simulink model "course_loop"  (R2019a)
settings: Solver=VariableStepAuto  StartTime=0.0  StopTime=300  RelTol=1e-3
undefined symbols (not defined in the file or in its folder): AP, trans_func
settings Model: Creator=nikhil  LastModifiedBy=VTOL_HYD

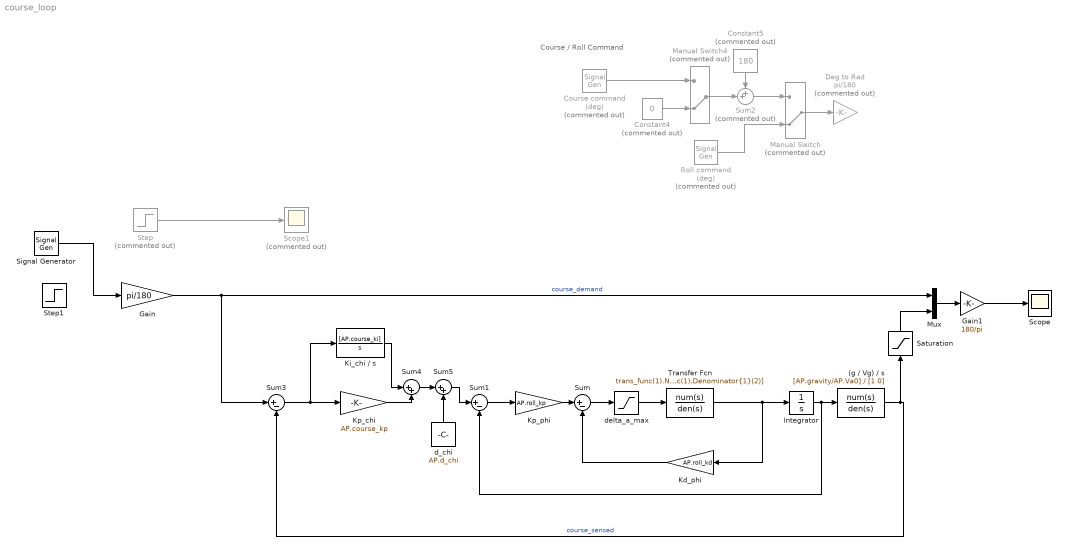
== system course_loop ==
  note: Course / Roll Command
  (g / Vg) / s : TransferFcn  Numerator=[AP.gravity/AP.Va0]  Denominator=[1 0]
  Constant4 : Constant  Commented=on  Value=0
  Constant5 : Constant  Commented=on  Value=180
  Course command (deg) : SignalGenerator  Commented=on  WaveForm=square  Amplitude=45  Frequency=.02
  Deg to Rad : Gain  Commented=on  Gain=pi/180
  Gain : Gain  Gain=pi/180
  Gain1 : Gain  Gain=180/pi
  Integrator : Integrator
  Kd_phi : Gain  Gain=AP.roll_kd
  Ki_chi / s : TransferFcn  Numerator=[AP.course_ki]  Denominator=[1 0]
  Kp_chi : Gain  Gain=AP.course_kp
  Kp_phi : Gain  Gain=AP.roll_kp
  Manual Switch : ManualSwitch  Commented=on  CurrentSetting=0
  Manual Switch4 : ManualSwitch  Commented=on  CurrentSetting=0
  Mux : Mux  Inputs=2
  Roll command (deg) : SignalGenerator  Commented=on  Amplitude=180  Frequency=0.1
  Saturation : Saturate  UpperLimit=7  LowerLimit=-7
  Scope : Scope
  Scope1 : Scope  Commented=on
  Signal Generator : SignalGenerator  Amplitude=110  Frequency=.09  Units=rad/sec
  Step : Step  Commented=on  Time=8  After=25  SampleTime=0
  Step1 : Step  After=200  SampleTime=5
  Sum : Sum  Inputs=|+-
  Sum1 : Sum  Inputs=|+-
  Sum2 : Sum  Commented=on  Inputs=++|
  Sum3 : Sum  Inputs=|+-
  Sum4 : Sum  Inputs=|++
  Sum5 : Sum  Inputs=|++
  Transfer Fcn : TransferFcn  Numerator=trans_func(1).Numerator{1}  Denominator=[trans_func(1).Denominator{1}(1), trans_func(1).Denominator{1}(2)]
  d_chi : Constant  Value=AP.d_chi
  delta_a_max : Saturate  UpperLimit=0.785  LowerLimit=-.785
  wires:
  Transfer Fcn/1 -> Kd_phi/1, Integrator/1
  Kd_phi/1 -> Sum/2
  Gain/1 -> Sum3/1, Mux/1  "course_demand"
  Sum1/1 -> Kp_phi/1
  Kp_phi/1 -> Sum/1
  (g / Vg) / s/1 -> Sum3/2, Saturation/1  "course_sensed"
  Sum3/1 -> Ki_chi / s/1, Kp_chi/1
  Ki_chi / s/1 -> Sum4/1
  Kp_chi/1 -> Sum4/2
  Step/1 -> Scope1/1
  Saturation/1 -> Mux/2
  Mux/1 -> Gain1/1
  Gain1/1 -> Scope/1
  Sum/1 -> delta_a_max/1
  delta_a_max/1 -> Transfer Fcn/1
  Integrator/1 -> (g / Vg) / s/1, Sum1/2
  d_chi/1 -> Sum5/2
  Sum4/1 -> Sum5/1
  Sum5/1 -> Sum1/1
  Signal Generator/1 -> Gain/1
  Constant5/1 -> Sum2/1
  Constant4/1 -> Manual Switch4/2
  Roll command (deg)/1 -> Manual Switch/2
  Manual Switch4/1 -> Sum2/2
  Manual Switch/1 -> Deg to Rad/1
  Course command (deg)/1 -> Manual Switch4/1
  Sum2/1 -> Manual Switch/1
